simulink model "SpeedgoatCANOpen2Buses100us"  (R2018b)
settings: Solver=FixedStepDiscrete  StartTime=0.0  StopTime=inf  FixedStep=0.0001  RelTol=1e-3  EnableMultiTasking=on
libraries: slrtlib x6, speedgoatlib_IO691 x5, simulink x3, dspstat3 x2, cstblocks x1
(part 1 of 2)
settings Model: DataDictionary=Trike_dictionary.sldd  SimulationMode=external  Creator=Venqo  LastModifiedBy=Venqo
settings SolverCC: ConcurrentTasks=on  AutoInsertRateTranBlk=on
settings DataIOCC: SaveFormat=StructureWithTime
settings OptimizationCC: BlockReduction=off  OptimizeBlockIOStorage=off  BufferReuse=off  GlobalBufferReuse=off  ExpressionFolding=off  LocalBlockOutputs=off  RollThreshold=10  OptimizeDataStoreBuffers=off  BusAssignmentInplaceUpdate=off
settings DebuggingCC: ParameterOverflowMsg=none
settings HardwareCC: ProdBitPerPointer=32  ProdBitPerSizeT=32  ProdBitPerPtrDiffT=32  ProdLargestAtomicFloat=None  ProdWordSize=32  ProdLongLongMode=on  ProdHWDeviceType=Generic->32-bit x86 compatible
settings SFSimCC: SimAnalyzeCustomCode=on
settings SFSimCC: SimCustomHeaderCode=|
  | #include "CANOpenSlave.h"
  | #include "CANOpenSlaveAPT.h"
settings SFSimCC: SimCustomInitializer=|
  | CANOpenSlave_ResetCommunication();
  | CANOpenSlave_ResetCommunication_APT();
settings SFSimCC: SimUserSources=|
  | CANOpenSlave.c
  | CANOpenSlaveAPT.c
settings RTWCC: SystemTargetFile=slrt.tlc  TemplateMakefile=slrt_default_tmf  Description=Simulink Real-Time  CodeExecutionProfiling=on  RTWCompilerOptimization=on
settings RTWCC: CustomHeaderCode=|
  | #include "CANOpenSlave.h"
  | #include "CANOpenSlaveAPT.h"
settings RTWCC: CustomSource=|
  | CANOpenSlave.c
  | CANOpenSlaveAPT.c
settings RTWCC: CustomInitializer=|
  | CANOpenSlave_ResetCommunication();
  | CANOpenSlave_ResetCommunication_APT();
settings SimulinkRealTimeCC: InferredTypesCompatibility=on  SupportVariableSizeSignals=on  PreserveStateflowLocalDataDimensions=off  RL32LogTETModifier=off  RL32LogBufSizeModifier=140000  xPCConcurrentTasks=on

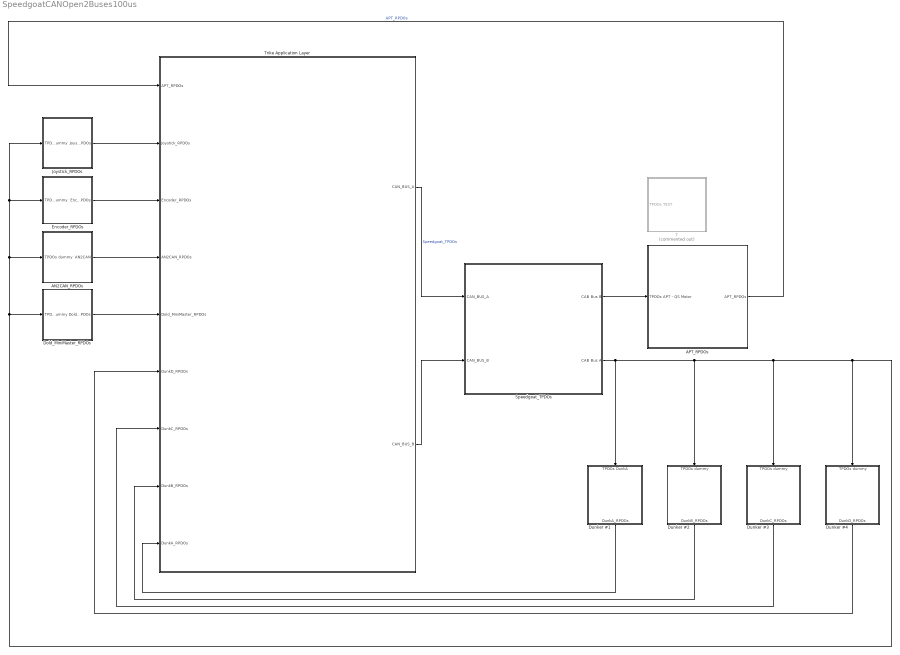
== system SpeedgoatCANOpen2Buses100us ==
  AN2CAN_RPDOs : Subsystem
      mask Display: image('Img\mcan_box_4xi.png');
  APT_RPDOs : Subsystem
      mask Display: image('Img\aptqsmotor.png');
  Dold_MiniMaster_RPDOs : Subsystem
      mask Display: image('C:\Users\Venqo\Desktop\SpeedGoat\Applications\Trike_git\Trike_SpeedGoat_algo\Img\dold - Copy.png');
  Dunker #1 : Subsystem
      mask Display: image('Img\dunk.png');
  Dunker #2 : Subsystem
      mask Display: image('Img\dunk.png');
  Dunker #3 : Subsystem
      mask Display: image('Img\dunk.png');
  Dunker #4 : Subsystem
      mask Display: image('Img\dunk.png');
  Encoder_RPDOs : Subsystem
      mask Display: image('Img\WDGA_Encoder.PNG');
  Joystick_RPDOs : Subsystem
      mask Display: image('Img\joystick.png');
  Speedgoat_TPDOs : Subsystem
      mask Display: image('Img\speedgoat.png');
  T : Subsystem  Commented=on
  Trike Application Layer : Subsystem
      mask Display: image('Img\trike.png');
  wires:
  Joystick_RPDOs/1(Joystick_RPDOs) -> Trike Application Layer/2(Joystick_RPDOs)
  Trike Application Layer/1(CAN_BUS_A) -> Speedgoat_TPDOs/1(CAN_BUS_A)  "Speedgoat_TPDOs"
  Dunker #1/1(DunkA_RPDOs) -> Trike Application Layer/9(DunkA_RPDOs)
  Encoder_RPDOs/1(Encoder_RPDOs) -> Trike Application Layer/3(Encoder_RPDOs)
  Dunker #2/1(DunkB_RPDOs) -> Trike Application Layer/8(DunkB_RPDOs)
  Dunker #3/1(DunkC_RPDOs) -> Trike Application Layer/7(DunkC_RPDOs)
  Dunker #4/1(DunkD_RPDOs) -> Trike Application Layer/6(DunkD_RPDOs)
  AN2CAN_RPDOs/1(AN2CAN) -> Trike Application Layer/4(AN2CAN_RPDOs)
  Speedgoat_TPDOs/1(CAB Bus B) -> APT_RPDOs/1("TPDOs APT - QS Motor ")
  APT_RPDOs/1(APT_RPDOs) -> Trike Application Layer/1(APT_RPDOs)  "APT_RPDOs"
  Trike Application Layer/2(CAN_BUS_B) -> Speedgoat_TPDOs/2(CAN_BUS_B)
  Dold_MiniMaster_RPDOs/1(Dold_RPDOs) -> Trike Application Layer/5(Dold_MiniMaster_RPDOs)
  Speedgoat_TPDOs/2("CAB Bus A ") -> Dold_MiniMaster_RPDOs/1(TPDOs dummy), Joystick_RPDOs/1(TPDOs dummy), Encoder_RPDOs/1(TPDOs dummy), AN2CAN_RPDOs/1(TPDOs dummy), Dunker #4/1(TPDOs dummy), Dunker #3/1(TPDOs dummy), Dunker #2/1(TPDOs dummy), Dunker #1/1(TPDOs DunkA)

== system SpeedgoatCANOpen2Buses100us/AN2CAN_RPDOs ==
  TPDOs dummy : Inport
  Bus Creator : BusCreator  Inputs=4  OutDataTypeStr=Bus: AN2CAN_conv
  "RPDOs from AN2CAN " : S-Function  InitFcn=try, set_param(gcb,'FunctionName','RPDOs_from_AN2CANConv'), end  FunctionName=RPDOs_from_AN2CANConv  SFunctionModules=RPDOs_from_AN2CANConv_wrapper  SFunctionDeploymentMode=off  EnableBusSupport=off  mask(S-Function Builder){}
      mask help: Simulink:masks:SFunctionBuilder_MD
      mask init:
      | val = [[.9  0.75 0.75 1 1 .9 .9 1]',[1 1 0.75 0.75 .9 .9 1 .9]'];try , sys = get_param(gcb,'SfunBuilderFcnName');if isempty(sys), sys = get_param(gcb,'FunctionName'); end,catch, sys = get_param(gcb,'FunctionName'); end
      settings: CopyFcn=set_param(gcbh,'LinkStatus','none')  PreSaveFcn=try, set_param(gcb,'FunctionName','RPDOs_from_AN2CANConv'), end  OpenFcn=sfunctionwizard(gcbh)
      mask Display: plot(val(:,1),val(:,2)),disp(sys), port_label('output',1,'Channel_AN1'), port_label('output',2,'Channel_AN2'), port_label('output',3,'Channel_AN3'), port_label('output',4,'Channel_AN4')
  AN2CAN : Outport  OutDataTypeStr=Bus: AN2CAN_conv
  wires:
  Bus Creator/1 -> AN2CAN/1
  "RPDOs from AN2CAN "/4 -> Bus Creator/4  "Channel_AN4"
  "RPDOs from AN2CAN "/3 -> Bus Creator/3  "Channel_AN3"
  "RPDOs from AN2CAN "/1 -> Bus Creator/1  "Channel_AN1"
  "RPDOs from AN2CAN "/2 -> Bus Creator/2  "Channel_AN2"

== system SpeedgoatCANOpen2Buses100us/APT_RPDOs ==
  "TPDOs APT - QS Motor " : Inport  OutDataTypeStr=Bus: Speedgoat_TPDOs
  Bus Creator : BusCreator  Inputs=8  OutDataTypeStr=Bus: APT_RPDOs
  Bus Selector : BusSelector  OutputSignals=APT_TPDO_ControlWord,APT_TPDO_PedalPosition,APT_TPDO_Heartbeat
  RPDOs from APT : S-Function  InitFcn=try, set_param(gcb,'FunctionName','RPDOs_from_APT'), end  FunctionName=RPDOs_from_APT  SFunctionModules=RPDOs_from_APT_wrapper  SFunctionDeploymentMode=off  EnableBusSupport=off  mask(S-Function Builder){}
      mask help: Simulink:masks:SFunctionBuilder_MD
      mask init: same as SpeedgoatCANOpen2Buses100us/AN2CAN_RPDOs/RPDOs from AN2CAN 
      settings: CopyFcn=set_param(gcbh,'LinkStatus','none')  PreSaveFcn=try, set_param(gcb,'FunctionName','RPDOs_from_APT'), end  OpenFcn=sfunctionwizard(gcbh)
      mask Display: plot(val(:,1),val(:,2)),disp(sys), port_label('output',1,'StatusWord'), port_label('output',2,'PhaseCurrent'), port_label('output',3,'Speed'), port_label('output',4,'BusVoltage'), port_label('output',5,'MotorTemp'), port_label('output',6,'APTTemp'), port_label('output',7,'ErrStatus'), port_label('output',8,'Direction')
  TPDOs from Speedgoat to APT : S-Function  InitFcn=try, set_param(gcb,'FunctionName','TPDOs_to_APT'), end  FunctionName=TPDOs_to_APT  SFunctionModules=TPDOs_to_APT_wrapper  SFunctionDeploymentMode=off  EnableBusSupport=off  mask(S-Function Builder){}
      mask help: Simulink:masks:SFunctionBuilder_MD
      mask init: same as SpeedgoatCANOpen2Buses100us/AN2CAN_RPDOs/RPDOs from AN2CAN 
      settings: CopyFcn=set_param(gcbh,'LinkStatus','none')  PreSaveFcn=try, set_param(gcb,'FunctionName','TPDOs_to_APT'), end  OpenFcn=sfunctionwizard(gcbh)
      mask Display: plot(val(:,1),val(:,2)),disp(sys), port_label('input',1,'APT_ControlWord'), port_label('input',2,'APT_PedalPosition'), port_label('input',3,'APT_HeartBeat')
  APT_RPDOs : Outport  OutDataTypeStr=Bus: APT_RPDOs
  wires:
  Bus Creator/1 -> APT_RPDOs/1
  RPDOs from APT/8 -> Bus Creator/8  "APT_Direction"
  RPDOs from APT/2 -> Bus Creator/2  "APT_PhaseCurrent"
  RPDOs from APT/6 -> Bus Creator/6  "APT_Temp"
  RPDOs from APT/3 -> Bus Creator/3  "APT_Speed"
  RPDOs from APT/1 -> Bus Creator/1  "APT_StatusWord"
  RPDOs from APT/5 -> Bus Creator/5  "APT_MotorTemp"
  RPDOs from APT/7 -> Bus Creator/7  "APT_ErrStatus"
  RPDOs from APT/4 -> Bus Creator/4  "APT_BusVoltage"
  "TPDOs APT - QS Motor "/1 -> Bus Selector/1
  Bus Selector/1 -> TPDOs from Speedgoat to APT/1  "<APT_TPDO_ControlWord>"
  Bus Selector/2 -> TPDOs from Speedgoat to APT/2  "<APT_TPDO_PedalPosition>"
  Bus Selector/3 -> TPDOs from Speedgoat to APT/3  "<APT_TPDO_Heartbeat>"

== system SpeedgoatCANOpen2Buses100us/Dold_MiniMaster_RPDOs ==
  TPDOs dummy : Inport
  Bus Creator : BusCreator  Inputs=1  OutDataTypeStr=Bus: Dold_RPDOs
  Constant : Constant  OutDataTypeStr=uint8
  Dold_RPDOs : Outport  OutDataTypeStr=Bus: Dold_RPDOs
  wires:
  Bus Creator/1 -> Dold_RPDOs/1
  Constant/1 -> Bus Creator/1  "Enable"

== system SpeedgoatCANOpen2Buses100us/Dunker #1 ==
  TPDOs DunkA : Inport  OutDataTypeStr=Bus: Speedgoat_TPDOs
  Bus Creator : BusCreator  Inputs=2  OutDataTypeStr=Bus: Dunk_RPDOs
  Bus Selector : BusSelector  OutputSignals=DunkA_TPDO_ClearError,DunkA_TPDO_DeviceMode,DunkA_TPDO_PowerEnable,DunkA_TPDO_BrakeCtrl,DunkA_TPDO_DesiredCurrent
  RPDOs from Dunker #1 : S-Function  InitFcn=try, set_param(gcb,'FunctionName','RPDOs_from_DunkA'), end  FunctionName=RPDOs_from_DunkA  SFunctionModules=RPDOs_from_DunkA_wrapper  SFunctionDeploymentMode=off  EnableBusSupport=off  mask(S-Function Builder){}
      mask help: Simulink:masks:SFunctionBuilder_MD
      mask init: same as SpeedgoatCANOpen2Buses100us/AN2CAN_RPDOs/RPDOs from AN2CAN 
      settings: CopyFcn=set_param(gcbh,'LinkStatus','none')  PreSaveFcn=try, set_param(gcb,'FunctionName','RPDOs_from_DunkA'), end  OpenFcn=sfunctionwizard(gcbh)
      mask Display: plot(val(:,1),val(:,2)),disp(sys), port_label('output',1,'ActualCurrent'), port_label('output',2,'ActualVelocity')
  TPDOs from Speedgoat to Dunker #1 : S-Function  InitFcn=try, set_param(gcb,'FunctionName','TPDOs_to_DunkA'), end  FunctionName=TPDOs_to_DunkA  SFunctionModules=TPDOs_to_DunkA_wrapper  SFunctionDeploymentMode=off  EnableBusSupport=off  mask(S-Function Builder){}
      mask help: Simulink:masks:SFunctionBuilder_MD
      mask init: same as SpeedgoatCANOpen2Buses100us/AN2CAN_RPDOs/RPDOs from AN2CAN 
      settings: CopyFcn=set_param(gcbh,'LinkStatus','none')  PreSaveFcn=try, set_param(gcb,'FunctionName','TPDOs_to_DunkA'), end  OpenFcn=sfunctionwizard(gcbh)
      mask Display: plot(val(:,1),val(:,2)),disp(sys), port_label('input',1,'ClearError'), port_label('input',2,'DeviceMode'), port_label('input',3,'PowerEnable'), port_label('input',4,'BrakeCtrl'), port_label('input',5,'DesiredCurrent')
  DunkA_RPDOs : Outport  OutDataTypeStr=Bus: Dunk_RPDOs
  wires:
  Bus Creator/1 -> DunkA_RPDOs/1
  RPDOs from Dunker #1/1 -> Bus Creator/1  "DunkA_ActualCurrent"
  RPDOs from Dunker #1/2 -> Bus Creator/2  "DunkA_ActualVelocity"
  Bus Selector/5 -> TPDOs from Speedgoat to Dunker #1/5  "<DunkA_TPDO_DesiredCurrent>"
  Bus Selector/1 -> TPDOs from Speedgoat to Dunker #1/1  "<DunkA_TPDO_ClearError>"
  Bus Selector/3 -> TPDOs from Speedgoat to Dunker #1/3  "<DunkA_TPDO_PowerEnable>"
  Bus Selector/4 -> TPDOs from Speedgoat to Dunker #1/4  "<DunkA_TPDO_BrakeCtrl>"
  Bus Selector/2 -> TPDOs from Speedgoat to Dunker #1/2  "<DunkA_TPDO_DeviceMode>"
  TPDOs DunkA/1 -> Bus Selector/1

== system SpeedgoatCANOpen2Buses100us/Dunker #2 ==
  TPDOs dummy : Inport  OutDataTypeStr=Bus: Speedgoat_TPDOs
  Bus Creator : BusCreator  Inputs=2  OutDataTypeStr=Bus: Dunk_RPDOs
  Bus Selector : BusSelector  OutputSignals=DunkB_TPDO_ClearError,DunkB_TPDO_DeviceMode,DunkB_TPDO_PowerEnable,DunkB_TPDO_BrakeCtrl,DunkB_TPDO_DesiredCurrent
  RPDOs from Dunker #1 : S-Function  InitFcn=try, set_param(gcb,'FunctionName','RPDOs_from_DunkB'), end  FunctionName=RPDOs_from_DunkB  SFunctionModules=RPDOs_from_DunkB_wrapper  SFunctionDeploymentMode=off  EnableBusSupport=off  mask(S-Function Builder){}
      mask help: Simulink:masks:SFunctionBuilder_MD
      mask init: same as SpeedgoatCANOpen2Buses100us/AN2CAN_RPDOs/RPDOs from AN2CAN 
      settings: CopyFcn=set_param(gcbh,'LinkStatus','none')  PreSaveFcn=try, set_param(gcb,'FunctionName','RPDOs_from_DunkB'), end  OpenFcn=sfunctionwizard(gcbh)
      mask Display: plot(val(:,1),val(:,2)),disp(sys), port_label('output',1,'ActualCurrent'), port_label('output',2,'ActualVelocity')
  TPDOs from Speedgoat to Dunker #1 : S-Function  InitFcn=try, set_param(gcb,'FunctionName','TPDOs_to_DunkB'), end  FunctionName=TPDOs_to_DunkB  SFunctionModules=TPDOs_to_DunkB_wrapper  SFunctionDeploymentMode=off  EnableBusSupport=off  mask(S-Function Builder){}
      mask help: Simulink:masks:SFunctionBuilder_MD
      mask init: same as SpeedgoatCANOpen2Buses100us/AN2CAN_RPDOs/RPDOs from AN2CAN 
      settings: CopyFcn=set_param(gcbh,'LinkStatus','none')  PreSaveFcn=try, set_param(gcb,'FunctionName','TPDOs_to_DunkB'), end  OpenFcn=sfunctionwizard(gcbh)
      mask Display: plot(val(:,1),val(:,2)),disp(sys), port_label('input',1,'ClearError'), port_label('input',2,'DeviceMode'), port_label('input',3,'PowerEnable'), port_label('input',4,'BrakeCtrl'), port_label('input',5,'DesiredCurrent')
  DunkB_RPDOs : Outport  OutDataTypeStr=Bus: Dunk_RPDOs
  wires:
  TPDOs dummy/1 -> Bus Selector/1
  Bus Selector/2 -> TPDOs from Speedgoat to Dunker #1/2  "<DunkB_TPDO_DeviceMode>"
  Bus Selector/4 -> TPDOs from Speedgoat to Dunker #1/4  "<DunkB_TPDO_BrakeCtrl>"
  Bus Selector/3 -> TPDOs from Speedgoat to Dunker #1/3  "<DunkB_TPDO_PowerEnable>"
  Bus Selector/1 -> TPDOs from Speedgoat to Dunker #1/1  "<DunkB_TPDO_ClearError>"
  Bus Selector/5 -> TPDOs from Speedgoat to Dunker #1/5  "<DunkB_TPDO_DesiredCurrent>"
  RPDOs from Dunker #1/2 -> Bus Creator/2  "DunkB_ActualVelocity"
  RPDOs from Dunker #1/1 -> Bus Creator/1  "DunkB_ActualCurrent"
  Bus Creator/1 -> DunkB_RPDOs/1

== system SpeedgoatCANOpen2Buses100us/Dunker #3 ==
  TPDOs dummy : Inport  OutDataTypeStr=Bus: Speedgoat_TPDOs
  Bus Creator : BusCreator  Inputs=2  OutDataTypeStr=Bus: Dunk_RPDOs
  Bus Selector : BusSelector  OutputSignals=DunkC_TPDO_ClearError,DunkC_TPDO_DeviceMode,DunkC_TPDO_PowerEnable,DunkC_TPDO_BrakeCtrl,DunkC_TPDO_DesiredCurrent
  Gain : Gain  Gain=-1
  RPDOs from Dunker #1 : S-Function  InitFcn=try, set_param(gcb,'FunctionName','RPDOs_from_DunkC'), end  FunctionName=RPDOs_from_DunkC  SFunctionModules=RPDOs_from_DunkC_wrapper  SFunctionDeploymentMode=off  EnableBusSupport=off  mask(S-Function Builder){}
      mask help: Simulink:masks:SFunctionBuilder_MD
      mask init: same as SpeedgoatCANOpen2Buses100us/AN2CAN_RPDOs/RPDOs from AN2CAN 
      settings: CopyFcn=set_param(gcbh,'LinkStatus','none')  PreSaveFcn=try, set_param(gcb,'FunctionName','RPDOs_from_DunkC'), end  OpenFcn=sfunctionwizard(gcbh)
      mask Display: plot(val(:,1),val(:,2)),disp(sys), port_label('output',1,'ActualCurrent'), port_label('output',2,'ActualVelocity')
  TPDOs from Speedgoat to Dunker #1 : S-Function  InitFcn=try, set_param(gcb,'FunctionName','TPDOs_to_DunkC'), end  FunctionName=TPDOs_to_DunkC  SFunctionModules=TPDOs_to_DunkC_wrapper  SFunctionDeploymentMode=off  EnableBusSupport=off  mask(S-Function Builder){}
      mask help: Simulink:masks:SFunctionBuilder_MD
      mask init: same as SpeedgoatCANOpen2Buses100us/AN2CAN_RPDOs/RPDOs from AN2CAN 
      settings: CopyFcn=set_param(gcbh,'LinkStatus','none')  PreSaveFcn=try, set_param(gcb,'FunctionName','TPDOs_to_DunkC'), end  OpenFcn=sfunctionwizard(gcbh)
      mask Display: plot(val(:,1),val(:,2)),disp(sys), port_label('input',1,'ClearError'), port_label('input',2,'DeviceMode'), port_label('input',3,'PowerEnable'), port_label('input',4,'BrakeCtrl'), port_label('input',5,'DesiredCurrent')
  Terminator : Terminator
  DunkC_RPDOs : Outport  OutDataTypeStr=Bus: Dunk_RPDOs
  wires:
  Bus Creator/1 -> DunkC_RPDOs/1
  RPDOs from Dunker #1/1 -> Gain/1, Bus Creator/1  "DunkC_ActualCurrent"
  RPDOs from Dunker #1/2 -> Bus Creator/2  "DunkC_ActualVelocity"
  Bus Selector/5 -> TPDOs from Speedgoat to Dunker #1/5  "<DunkC_TPDO_DesiredCurrent>"
  Bus Selector/1 -> TPDOs from Speedgoat to Dunker #1/1  "<DunkC_TPDO_ClearError>"
  Bus Selector/2 -> TPDOs from Speedgoat to Dunker #1/2  "<DunkC_TPDO_DeviceMode>"
  Bus Selector/4 -> TPDOs from Speedgoat to Dunker #1/4  "<DunkC_TPDO_BrakeCtrl>"
  Bus Selector/3 -> TPDOs from Speedgoat to Dunker #1/3  "<DunkC_TPDO_PowerEnable>"
  TPDOs dummy/1 -> Bus Selector/1
  Gain/1 -> Terminator/1  "DunkC_ActualCurrent_Inv"

== system SpeedgoatCANOpen2Buses100us/Dunker #4 ==
  TPDOs dummy : Inport  OutDataTypeStr=Bus: Speedgoat_TPDOs
  Bus Creator : BusCreator  Inputs=2  OutDataTypeStr=Bus: Dunk_RPDOs
  Bus Selector : BusSelector  OutputSignals=DunkD_TPDO_ClearError,DunkD_TPDO_DeviceMode,DunkD_TPDO_PowerEnable,DunkD_TPDO_BrakeCtrl,DunkD_TPDO_DesiredCurrent
  RPDOs from Dunker #1 : S-Function  InitFcn=try, set_param(gcb,'FunctionName','RPDOs_from_DunkD'), end  FunctionName=RPDOs_from_DunkD  SFunctionModules=RPDOs_from_DunkD_wrapper  SFunctionDeploymentMode=off  EnableBusSupport=off  mask(S-Function Builder){}
      mask help: Simulink:masks:SFunctionBuilder_MD
      mask init: same as SpeedgoatCANOpen2Buses100us/AN2CAN_RPDOs/RPDOs from AN2CAN 
      settings: CopyFcn=set_param(gcbh,'LinkStatus','none')  PreSaveFcn=try, set_param(gcb,'FunctionName','RPDOs_from_DunkD'), end  OpenFcn=sfunctionwizard(gcbh)
      mask Display: plot(val(:,1),val(:,2)),disp(sys), port_label('output',1,'ActualCurrent'), port_label('output',2,'ActualVelocity')
  TPDOs from Speedgoat to Dunker #1 : S-Function  InitFcn=try, set_param(gcb,'FunctionName','TPDOs_to_DunkD'), end  FunctionName=TPDOs_to_DunkD  SFunctionModules=TPDOs_to_DunkD_wrapper  SFunctionDeploymentMode=off  EnableBusSupport=off  mask(S-Function Builder){}
      mask help: Simulink:masks:SFunctionBuilder_MD
      mask init: same as SpeedgoatCANOpen2Buses100us/AN2CAN_RPDOs/RPDOs from AN2CAN 
      settings: CopyFcn=set_param(gcbh,'LinkStatus','none')  PreSaveFcn=try, set_param(gcb,'FunctionName','TPDOs_to_DunkD'), end  OpenFcn=sfunctionwizard(gcbh)
      mask Display: plot(val(:,1),val(:,2)),disp(sys), port_label('input',1,'ClearError'), port_label('input',2,'DeviceMode'), port_label('input',3,'PowerEnable'), port_label('input',4,'BrakeCtrl'), port_label('input',5,'DesiredCurrent')
  DunkD_RPDOs : Outport  OutDataTypeStr=Bus: Dunk_RPDOs
  wires:
  TPDOs dummy/1 -> Bus Selector/1
  Bus Selector/2 -> TPDOs from Speedgoat to Dunker #1/2  "<DunkD_TPDO_DeviceMode>"
  Bus Selector/4 -> TPDOs from Speedgoat to Dunker #1/4  "<DunkD_TPDO_BrakeCtrl>"
  Bus Selector/3 -> TPDOs from Speedgoat to Dunker #1/3  "<DunkD_TPDO_PowerEnable>"
  Bus Selector/1 -> TPDOs from Speedgoat to Dunker #1/1  "<DunkD_TPDO_ClearError>"
  Bus Selector/5 -> TPDOs from Speedgoat to Dunker #1/5  "<DunkD_TPDO_DesiredCurrent>"
  RPDOs from Dunker #1/2 -> Bus Creator/2  "DunkD_ActualVelocity"
  RPDOs from Dunker #1/1 -> Bus Creator/1  "DunkD_ActualCurrent"
  Bus Creator/1 -> DunkD_RPDOs/1

== system SpeedgoatCANOpen2Buses100us/Encoder_RPDOs ==
  TPDOs dummy : Inport
  Bus Creator : BusCreator  Inputs=2  OutDataTypeStr=Bus: Encoder_RPDOs
  RPDOs from Encoder : S-Function  InitFcn=try, set_param(gcb,'FunctionName','RPDOs_from_Encoder'), end  FunctionName=RPDOs_from_Encoder  SFunctionModules=RPDOs_from_Encoder_wrapper  SFunctionDeploymentMode=off  EnableBusSupport=off  mask(S-Function Builder){}
      mask help: Simulink:masks:SFunctionBuilder_MD
      mask init: same as SpeedgoatCANOpen2Buses100us/AN2CAN_RPDOs/RPDOs from AN2CAN 
      settings: CopyFcn=set_param(gcbh,'LinkStatus','none')  PreSaveFcn=try, set_param(gcb,'FunctionName','RPDOs_from_Encoder'), end  OpenFcn=sfunctionwizard(gcbh)
      mask Display: plot(val(:,1),val(:,2)),disp(sys), port_label('output',1,'Encoder_Actual_Position'), port_label('output',2,'Encoder_Stored_Position')
  Encoder_RPDOs : Outport  OutDataTypeStr=Bus: Encoder_RPDOs
  wires:
  RPDOs from Encoder/1 -> Bus Creator/1  "Encoder_Actual_Position"
  RPDOs from Encoder/2 -> Bus Creator/2  "Encoder_Stored_Position"
  Bus Creator/1 -> Encoder_RPDOs/1

== system SpeedgoatCANOpen2Buses100us/Joystick_RPDOs ==
  TPDOs dummy : Inport
  Bus Creator : BusCreator  Inputs=3  OutDataTypeStr=Bus: Joystick_RPDOs
  RPDOs from Joystick : S-Function  InitFcn=try, set_param(gcb,'FunctionName','RPDOs_from_Joystick'), end  FunctionName=RPDOs_from_Joystick  SFunctionModules=RPDOs_from_Joystick_wrapper  SFunctionDeploymentMode=off  EnableBusSupport=off  mask(S-Function Builder){}
      mask help: Simulink:masks:SFunctionBuilder_MD
      mask init: same as SpeedgoatCANOpen2Buses100us/AN2CAN_RPDOs/RPDOs from AN2CAN 
      settings: CopyFcn=set_param(gcbh,'LinkStatus','none')  PreSaveFcn=try, set_param(gcb,'FunctionName','RPDOs_from_Joystick'), end  OpenFcn=sfunctionwizard(gcbh)
      mask Display: plot(val(:,1),val(:,2)),disp(sys), port_label('output',1,'ButtonsStatus'), port_label('output',2,'LongCmd'), port_label('output',3,'LatCmd')
  Joystick_RPDOs : Outport  OutDataTypeStr=Bus: Joystick_RPDOs
  wires:
  RPDOs from Joystick/3 -> Bus Creator/3  "Joystick_LatCmd"
  RPDOs from Joystick/2 -> Bus Creator/2  "Joystick_LongCmd"
  RPDOs from Joystick/1 -> Bus Creator/1  "Joystick_ButtonsStatus"
  Bus Creator/1 -> Joystick_RPDOs/1

== system SpeedgoatCANOpen2Buses100us/Speedgoat_TPDOs ==
  CAN_BUS_A : Inport  OutDataTypeStr=Bus: CAN_BUS_A
  CAN_BUS_B : Inport  Port=2  OutDataTypeStr=Bus: CAN_BUS_B
  CAN Bus Communication : Subsystem
  Subsystem : Subsystem
  CAB Bus B : Outport  OutDataTypeStr=Bus: Speedgoat_TPDOs
  "CAB Bus A " : Outport  Port=2  OutDataTypeStr=Bus: Speedgoat_TPDOs
  wires:
  Subsystem/1(SpeedGoat) -> "CAB Bus A "/1, CAB Bus B/1
  CAN_BUS_B/1 -> Subsystem/2(CAN_BUS_B)
  CAN_BUS_A/1 -> Subsystem/1(CAN_BUS_A)

== system SpeedgoatCANOpen2Buses100us/T ==
  TPDOs TEST : Inport  OutDataTypeStr=Bus: Speedgoat_TPDOs
  Bus Selector : BusSelector  OutputSignals=AN_01,AN_02,AN_03,AN_04
  TPDOs from Speedgoat to Dunker #1 : S-Function  InitFcn=try, set_param(gcb,'FunctionName','TPDOs_TEST'), end  FunctionName=TPDOs_TEST  SFunctionModules=TPDOs_TEST_wrapper  SFunctionDeploymentMode=off  EnableBusSupport=off  mask(S-Function Builder){}
      mask help: Simulink:masks:SFunctionBuilder_MD
      mask init: same as SpeedgoatCANOpen2Buses100us/AN2CAN_RPDOs/RPDOs from AN2CAN 
      settings: CopyFcn=set_param(gcbh,'LinkStatus','none')  PreSaveFcn=try, set_param(gcb,'FunctionName','TPDOs_TEST'), end  OpenFcn=sfunctionwizard(gcbh)
      mask Display: plot(val(:,1),val(:,2)),disp(sys), port_label('input',1,'AN1'), port_label('input',2,'AN2'), port_label('input',3,'AN3'), port_label('input',4,'AN4')
  wires:
  Bus Selector/1 -> TPDOs from Speedgoat to Dunker #1/1  "<AN_01>"
  Bus Selector/3 -> TPDOs from Speedgoat to Dunker #1/3  "<AN_03>"
  Bus Selector/4 -> TPDOs from Speedgoat to Dunker #1/4  "<AN_04>"
  Bus Selector/2 -> TPDOs from Speedgoat to Dunker #1/2  "<AN_02>"
  TPDOs TEST/1 -> Bus Selector/1

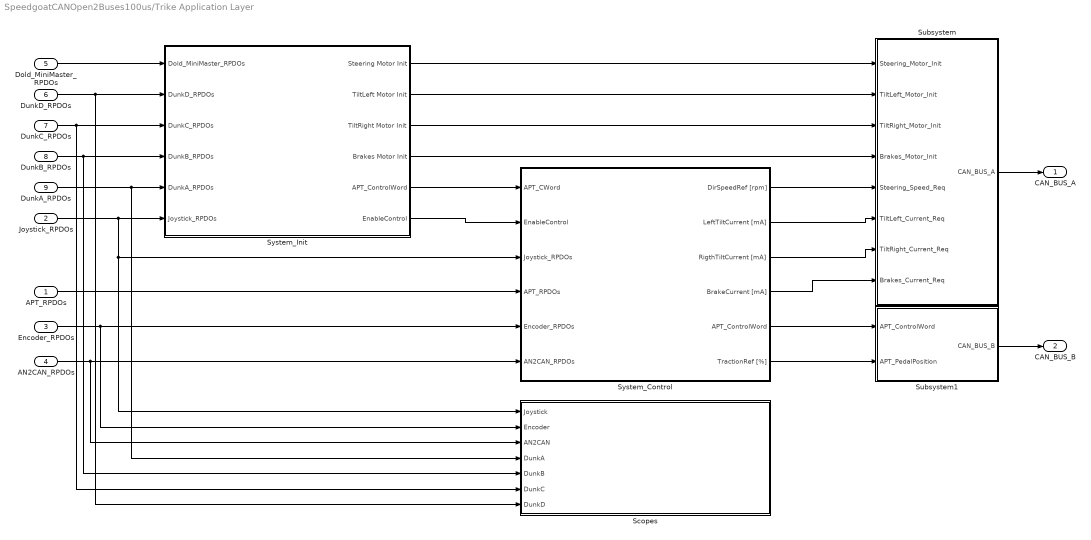
== system SpeedgoatCANOpen2Buses100us/Trike Application Layer ==
  APT_RPDOs : Inport  OutDataTypeStr=Bus: APT_RPDOs
  Joystick_RPDOs : Inport  Port=2  OutDataTypeStr=Bus: Joystick_RPDOs
  Encoder_RPDOs : Inport  Port=3  OutDataTypeStr=Bus: Encoder_RPDOs
  AN2CAN_RPDOs : Inport  Port=4  OutDataTypeStr=Bus: AN2CAN_conv
  Dold_MiniMaster_RPDOs : Inport  Port=5  OutDataTypeStr=Bus: Dold_RPDOs
  DunkD_RPDOs : Inport  Port=6  OutDataTypeStr=Bus: Dunk_RPDOs
  DunkC_RPDOs : Inport  Port=7  OutDataTypeStr=Bus: Dunk_RPDOs
  DunkB_RPDOs : Inport  Port=8  OutDataTypeStr=Bus: Dunk_RPDOs
  DunkA_RPDOs : Inport  Port=9  OutDataTypeStr=Bus: Dunk_RPDOs
  Scopes : Subsystem
  Subsystem : Subsystem
  Subsystem1 : Subsystem
  System_Control : Subsystem
  System_Init : Subsystem
  CAN_BUS_A : Outport  OutDataTypeStr=Bus: CAN_BUS_A
  CAN_BUS_B : Outport  Port=2  OutDataTypeStr=Bus: CAN_BUS_B
  wires:
  Subsystem/1(CAN_BUS_A) -> CAN_BUS_A/1
  System_Control/1(DirSpeedRef [rpm]) -> Subsystem/5(Steering_Speed_Req)
  System_Control/2(LeftTiltCurrent [mA]) -> Subsystem/6(TiltLeft_Current_Req)
  System_Control/3(RigthTiltCurrent [mA]) -> Subsystem/7(TiltRight_Current_Req)
  System_Control/4(BrakeCurrent [mA]) -> Subsystem/8(Brakes_Current_Req)
  Subsystem1/1(CAN_BUS_B) -> CAN_BUS_B/1
  System_Control/6(TractionRef [%]) -> Subsystem1/2(APT_PedalPosition)
  DunkA_RPDOs/1 -> System_Init/5(DunkA_RPDOs), Scopes/4(DunkA)
  DunkB_RPDOs/1 -> System_Init/4(DunkB_RPDOs), Scopes/5(DunkB)
  DunkC_RPDOs/1 -> System_Init/3(DunkC_RPDOs), Scopes/6(DunkC)
  DunkD_RPDOs/1 -> Scopes/7(DunkD), System_Init/2(DunkD_RPDOs)
  System_Init/1(Steering Motor Init) -> Subsystem/1(Steering_Motor_Init)
  System_Init/2(TiltLeft Motor Init) -> Subsystem/2(TiltLeft_Motor_Init)
  System_Init/3(TiltRight Motor Init) -> Subsystem/3(TiltRight_Motor_Init)
  System_Init/4(Brakes Motor Init) -> Subsystem/4(Brakes_Motor_Init)
  System_Control/5(APT_ControlWord) -> Subsystem1/1(APT_ControlWord)
  AN2CAN_RPDOs/1 -> Scopes/3(AN2CAN), System_Control/6(AN2CAN_RPDOs)
  Encoder_RPDOs/1 -> Scopes/2(Encoder), System_Control/5(Encoder_RPDOs)
  APT_RPDOs/1 -> System_Control/4(APT_RPDOs)
  System_Init/6(EnableControl) -> System_Control/2(EnableControl)
  Joystick_RPDOs/1 -> System_Init/6(Joystick_RPDOs), Scopes/1(Joystick), System_Control/3(Joystick_RPDOs)
  System_Init/5(APT_ControlWord) -> System_Control/1(APT_CWord)
  Dold_MiniMaster_RPDOs/1 -> System_Init/1(Dold_MiniMaster_RPDOs)

== system SpeedgoatCANOpen2Buses100us/Speedgoat_TPDOs/CAN Bus Communication ==
  "CAN Setup " : speedgoatlib_IO691/CAN Setup   moduletype=IO691  id=1  pciSlot=-1  chn1=CAN (HS)  chn2=CAN (HS)  chn3=Disabled  chn4=Disabled  initStruct=[]  termStruct=[]  ArbitrationbdrChn1=500 kBaud  ArbitrationManbdrChn1=[2,16,63,16]  FdbdrChn1=5.0 MBaud  FdManbdrChn1=[2,2,5,2]  ArbitrationbdrChn2=500 kBaud  ArbitrationManbdrChn2=[2,16,63,16]  FdbdrChn2=5.0 MBaud  FdManbdrChn2=[2,2,5,2]  ArbitrationbdrChn3=1.0 MBaud  ArbitrationManbdrChn3=[2,8,31,8]  FdbdrChn3=5.0 MBaud  FdManbdrChn3=[2,2,5,2]  ArbitrationbdrChn4=1.0 MBaud  ArbitrationManbdrChn4=[2,8,31,8]  FdbdrChn4=5.0 MBaud  FdManbdrChn4=[2,2,5,2]  moduleInitValues=[691 1 -1 -1]
      settings: SourceProductName=Simulink Real-Time: Speedgoat Library
  CANOpen Slave Protocol Stack - CAN Bus #1 (A) : Subsystem  mask{Ts=0.0001}
      mask prompts: Ts "Sample Time (s)"
      mask Display: disp('CANOpen Slave Stack')
  CANOpen Slave Protocol Stack - CAN Bus #2 (B) : Subsystem  mask{Ts=0.0001}
      mask prompts: Ts "Sample Time (s)"
      mask Display: disp('CANOpen Slave Stack')

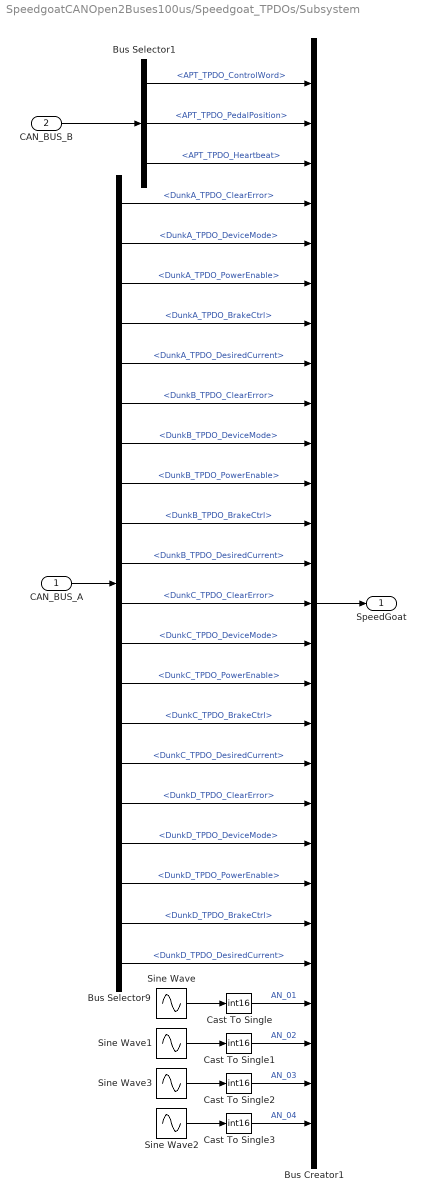
== system SpeedgoatCANOpen2Buses100us/Speedgoat_TPDOs/Subsystem ==
  CAN_BUS_A : Inport  OutDataTypeStr=Bus: CAN_BUS_A
  CAN_BUS_B : Inport  Port=2  OutDataTypeStr=Bus: CAN_BUS_B
  Bus Creator1 : BusCreator  Inputs=27  OutDataTypeStr=Bus: Speedgoat_TPDOs
  Bus Selector1 : BusSelector  OutputSignals=APT_TPDO_ControlWord,APT_TPDO_PedalPosition,APT_TPDO_Heartbeat
  Bus Selector9 : BusSelector  OutputSignals=DunkA_TPDO_ClearError,DunkA_TPDO_DeviceMode,DunkA_TPDO_PowerEnable,DunkA_TPDO_BrakeCtrl,DunkA_TPDO_DesiredCurrent,DunkB_TPDO_ClearError,DunkB_TPDO_DeviceMode,DunkB_TPDO_PowerEnable,DunkB_TPDO_BrakeCtrl,DunkB_TPDO_DesiredCurrent,DunkC_TPDO_ClearError,DunkC_TPDO_DeviceMode,DunkC_TPDO_PowerEnable,DunkC_TPDO_BrakeCtrl,DunkC_TPDO_DesiredCurrent,DunkD_TPDO_ClearError,DunkD_TPDO_DeviceMode,DunkD_TPDO_PowerEnable,DunkD_TPDO_BrakeCtrl,DunkD_TPDO_DesiredCurrent
  Cast To Single{,1..3} (4 alike) : DataTypeConversion  OutDataTypeStr=int16
  Sine Wave{,1..3} (4 alike) : Sin  Amplitude=5000  Bias=2500  Frequency=4  SampleTime=0
  SpeedGoat : Outport  OutDataTypeStr=Bus: Speedgoat_TPDOs
  wires:
  Bus Creator1/1 -> SpeedGoat/1
  CAN_BUS_A/1 -> Bus Selector9/1
  CAN_BUS_B/1 -> Bus Selector1/1
  Bus Selector1/1 -> Bus Creator1/1  "<APT_TPDO_ControlWord>"
  Bus Selector1/2 -> Bus Creator1/2  "<APT_TPDO_PedalPosition>"
  Bus Selector1/3 -> Bus Creator1/3  "<APT_TPDO_Heartbeat>"
  Bus Selector9/1 -> Bus Creator1/4  "<DunkA_TPDO_ClearError>"
  Bus Selector9/2 -> Bus Creator1/5  "<DunkA_TPDO_DeviceMode>"
  Bus Selector9/3 -> Bus Creator1/6  "<DunkA_TPDO_PowerEnable>"
  Bus Selector9/4 -> Bus Creator1/7  "<DunkA_TPDO_BrakeCtrl>"
  Bus Selector9/5 -> Bus Creator1/8  "<DunkA_TPDO_DesiredCurrent>"
  Bus Selector9/6 -> Bus Creator1/9  "<DunkB_TPDO_ClearError>"
  Bus Selector9/7 -> Bus Creator1/10  "<DunkB_TPDO_DeviceMode>"
  Bus Selector9/8 -> Bus Creator1/11  "<DunkB_TPDO_PowerEnable>"
  Bus Selector9/9 -> Bus Creator1/12  "<DunkB_TPDO_BrakeCtrl>"
  Bus Selector9/10 -> Bus Creator1/13  "<DunkB_TPDO_DesiredCurrent>"
  Bus Selector9/11 -> Bus Creator1/14  "<DunkC_TPDO_ClearError>"
  Bus Selector9/12 -> Bus Creator1/15  "<DunkC_TPDO_DeviceMode>"
  Bus Selector9/13 -> Bus Creator1/16  "<DunkC_TPDO_PowerEnable>"
  Bus Selector9/14 -> Bus Creator1/17  "<DunkC_TPDO_BrakeCtrl>"
  Bus Selector9/15 -> Bus Creator1/18  "<DunkC_TPDO_DesiredCurrent>"
  Bus Selector9/16 -> Bus Creator1/19  "<DunkD_TPDO_ClearError>"
  Bus Selector9/17 -> Bus Creator1/20  "<DunkD_TPDO_DeviceMode>"
  Bus Selector9/18 -> Bus Creator1/21  "<DunkD_TPDO_PowerEnable>"
  Bus Selector9/19 -> Bus Creator1/22  "<DunkD_TPDO_BrakeCtrl>"
  Bus Selector9/20 -> Bus Creator1/23  "<DunkD_TPDO_DesiredCurrent>"
  Sine Wave/1 -> Cast To Single/1
  Sine Wave1/1 -> Cast To Single1/1
  Sine Wave2/1 -> Cast To Single3/1
  Sine Wave3/1 -> Cast To Single2/1
  Cast To Single/1 -> Bus Creator1/24  "AN_01"
  Cast To Single1/1 -> Bus Creator1/25  "AN_02"
  Cast To Single2/1 -> Bus Creator1/26  "AN_03"
  Cast To Single3/1 -> Bus Creator1/27  "AN_04"

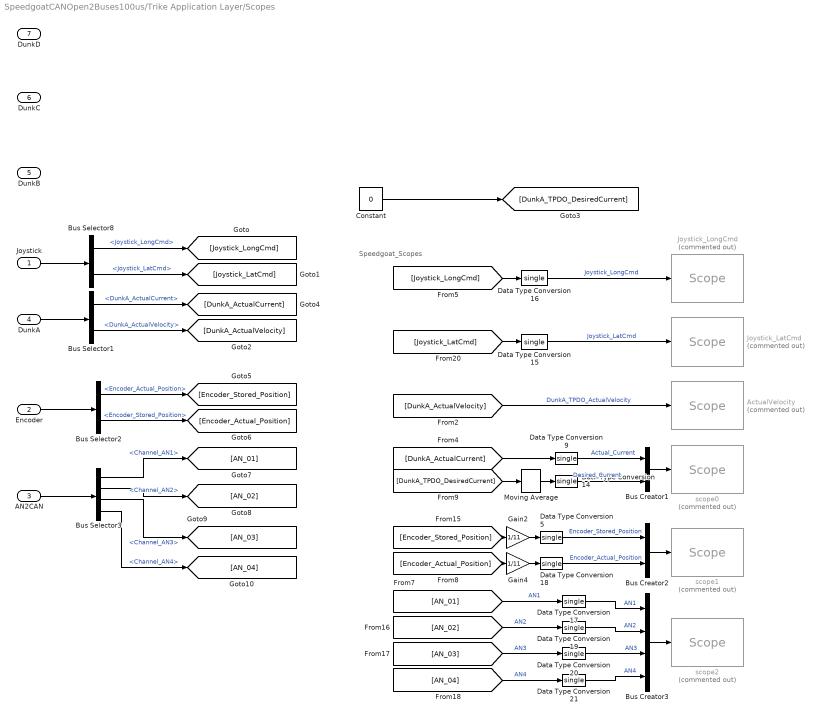
== system SpeedgoatCANOpen2Buses100us/Trike Application Layer/Scopes ==
  note: Speedgoat_Scopes
  Joystick : Inport
  Encoder : Inport  Port=2
  AN2CAN : Inport  Port=3
  DunkA : Inport  Port=4
  DunkB : Inport  Port=5
  DunkC : Inport  Port=6
  DunkD : Inport  Port=7
  ActualVelocity : slrtlib/Displays and Logging/Scope   Commented=on  scopeno=3  scopetype=Target  autostart=on  viewmode=Graphical sliding  formatstr='%15.6f'  grid=on  ylimits=[-3000,3000]  nosamples=30000  noprepostsamples=0  interleave=1  triggermode=FreeRun  triggersignal=1  trigsignalfromport=off  triggerlevel=0.0  triggerslope=Rising  triggerscope=1  triggersample=0  filename=data.dat  mode=Lazy  writesize=512  autorestart=off  dynamicfilemode=off  maxwritefilesize=512*1024^2
  Bus Creator1 : BusCreator  Inputs=2
  Bus Creator2 : BusCreator  Inputs=2
  Bus Creator3 : BusCreator  Inputs=4
  Bus Selector1 : BusSelector  OutputSignals=DunkA_ActualCurrent,DunkA_ActualVelocity
  Bus Selector2 : BusSelector  OutputSignals=Encoder_Actual_Position,Encoder_Stored_Position
  Bus Selector3 : BusSelector  OutputSignals=Channel_AN1,Channel_AN2,Channel_AN3,Channel_AN4
  Bus Selector8 : BusSelector  OutputSignals=Joystick_LongCmd,Joystick_LatCmd
  Constant : Constant  Value=0
  Data Type Conversion{5,9,14..21} (10 alike) : DataTypeConversion  OutDataTypeStr=single
  Gain2 : Gain  Gain=1/11
  Gain4 : Gain  Gain=1/11
  Joystick_LatCmd : slrtlib/Displays and Logging/Scope   Commented=on  scopeno=2  scopetype=Target  autostart=on  viewmode=Graphical sliding  formatstr='%15.6f'  grid=on  ylimits=[-300,300]  nosamples=30000  noprepostsamples=0  interleave=1  triggermode=FreeRun  triggersignal=1  trigsignalfromport=off  triggerlevel=0.0  triggerslope=Rising  triggerscope=1  triggersample=0  filename=data.dat  mode=Lazy  writesize=512  autorestart=off  dynamicfilemode=off  maxwritefilesize=512*1024^2
  Joystick_LongCmd : slrtlib/Displays and Logging/Scope   Commented=on  scopeno=1  scopetype=Target  autostart=on  viewmode=Graphical sliding  formatstr='%15.6f'  grid=on  ylimits=[-300,300]  nosamples=30000  noprepostsamples=0  interleave=1  triggermode=FreeRun  triggersignal=1  trigsignalfromport=off  triggerlevel=0.0  triggerslope=Rising  triggerscope=1  triggersample=0  filename=data.dat  mode=Lazy  writesize=512  autorestart=off  dynamicfilemode=off  maxwritefilesize=512*1024^2
  Moving Average : dspstat3/Moving Average  Method=Sliding window  ForgettingFactorPort=off  SpecifyWindowLength=on  WindowLength=50  ForgettingFactor=0.9  SimulateUsing=Code generation
  scope0 : slrtlib/Displays and Logging/Scope   Commented=on  scopeno=4  scopetype=Target  autostart=on  viewmode=Graphical sliding  formatstr='%15.6f'  grid=on  ylimits=[-10000,10000]  nosamples=30000  noprepostsamples=0  interleave=1  triggermode=FreeRun  triggersignal=1  trigsignalfromport=off  triggerlevel=0.0  triggerslope=Rising  triggerscope=1  triggersample=0  filename=data.dat  mode=Lazy  writesize=512  autorestart=off  dynamicfilemode=off  maxwritefilesize=512*1024^2
  scope1 : slrtlib/Displays and Logging/Scope   Commented=on  scopeno=5  scopetype=Target  autostart=on  viewmode=Graphical sliding  formatstr='%15.6f'  grid=on  ylimits=[0,400]  nosamples=30000  noprepostsamples=0  interleave=1  triggermode=FreeRun  triggersignal=1  trigsignalfromport=off  triggerlevel=0.0  triggerslope=Rising  triggerscope=1  triggersample=0  filename=data.dat  mode=Lazy  writesize=512  autorestart=off  dynamicfilemode=off  maxwritefilesize=512*1024^2
  scope2 : slrtlib/Displays and Logging/Scope   Commented=on  scopeno=6  scopetype=Target  autostart=on  viewmode=Graphical sliding  formatstr='%15.6f'  grid=on  ylimits=[0,40000]  nosamples=30000  noprepostsamples=0  interleave=1  triggermode=FreeRun  triggersignal=1  trigsignalfromport=off  triggerlevel=0.0  triggerslope=Rising  triggerscope=1  triggersample=0  filename=data.dat  mode=Lazy  writesize=512  autorestart=off  dynamicfilemode=off  maxwritefilesize=512*1024^2
  wires:
  [Encoder_Actual_Position] -> Gain4/1
  [DunkA_TPDO_DesiredCurrent] -> Moving Average/1
  [Joystick_LatCmd] -> Data Type Conversion15/1
  [Joystick_LongCmd] -> Data Type Conversion16/1
  Data Type Conversion5/1 -> Bus Creator2/1  "Encoder_Stored_Position"
  Bus Selector3/3 -> [AN_03]  "<Channel_AN3>"
  [DunkA_ActualCurrent] -> Data Type Conversion9/1
  [AN_01] -> Data Type Conversion17/1  "AN1"
  Bus Creator2/1 -> scope1/1
  Bus Selector1/2 -> [DunkA_ActualVelocity]  "<DunkA_ActualVelocity>"
  Data Type Conversion15/1 -> Joystick_LatCmd/1  "Joystick_LatCmd"
  Constant/1 -> [DunkA_TPDO_DesiredCurrent]
  [AN_04] -> Data Type Conversion21/1  "AN4"
  Data Type Conversion9/1 -> Bus Creator1/1  "Actual_Current"
  [DunkA_ActualVelocity] -> ActualVelocity/1  "DunkA_TPDO_ActualVelocity"
  Gain4/1 -> Data Type Conversion18/1
  Data Type Conversion19/1 -> Bus Creator3/2  "AN2"
  Joystick/1 -> Bus Selector8/1
  Bus Selector1/1 -> [DunkA_ActualCurrent]  "<DunkA_ActualCurrent>"
  Data Type Conversion18/1 -> Bus Creator2/2  "Encoder_Actual_Position"
  Data Type Conversion14/1 -> Bus Creator1/2  "Desired_Current"
  [Encoder_Stored_Position] -> Gain2/1
  Data Type Conversion20/1 -> Bus Creator3/3  "AN3"
  Moving Average/1 -> Data Type Conversion14/1
  Encoder/1 -> Bus Selector2/1
  Bus Selector8/1 -> [Joystick_LongCmd]  "<Joystick_LongCmd>"
  [AN_03] -> Data Type Conversion20/1  "AN3"
  Bus Selector8/2 -> [Joystick_LatCmd]  "<Joystick_LatCmd>"
  Bus Selector2/2 -> [Encoder_Actual_Position]  "<Encoder_Stored_Position>"
  Data Type Conversion16/1 -> Joystick_LongCmd/1  "Joystick_LongCmd"
  Bus Creator3/1 -> scope2/1
  [AN_02] -> Data Type Conversion19/1  "AN2"
  Data Type Conversion17/1 -> Bus Creator3/1  "AN1"
  Gain2/1 -> Data Type Conversion5/1
  Data Type Conversion21/1 -> Bus Creator3/4  "AN4"
  Bus Creator1/1 -> scope0/1
  Bus Selector3/2 -> [AN_02]  "<Channel_AN2>"
  Bus Selector3/1 -> [AN_01]  "<Channel_AN1>"
  Bus Selector2/1 -> [Encoder_Stored_Position]  "<Encoder_Actual_Position>"
  Bus Selector3/4 -> [AN_04]  "<Channel_AN4>"
  AN2CAN/1 -> Bus Selector3/1
  DunkA/1 -> Bus Selector1/1

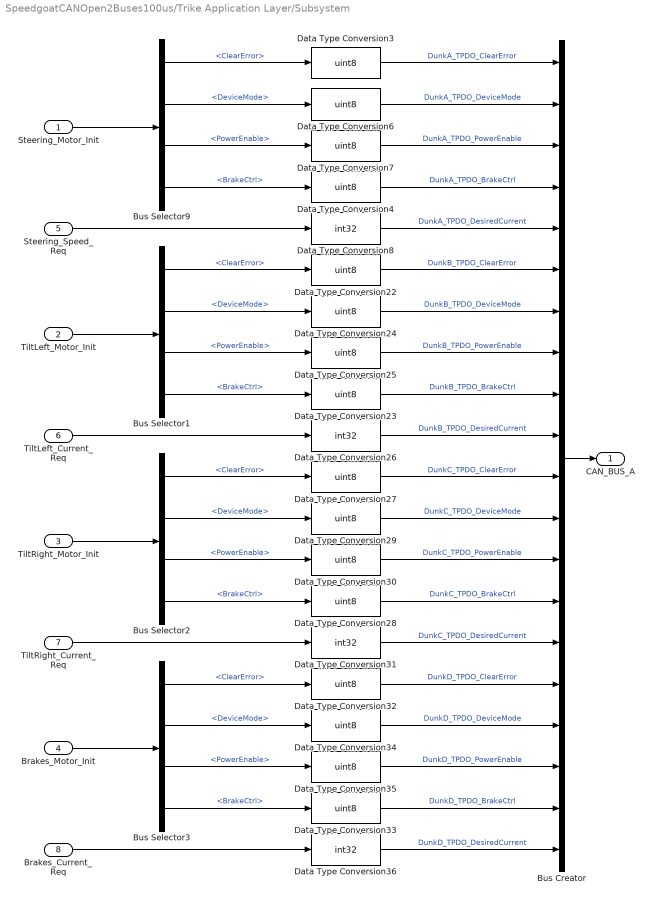
== system SpeedgoatCANOpen2Buses100us/Trike Application Layer/Subsystem ==
  Steering_Motor_Init : Inport  OutDataTypeStr=Bus: Dunk_Init_TPDOs
  TiltLeft_Motor_Init : Inport  Port=2  OutDataTypeStr=Bus: Dunk_Init_TPDOs
  TiltRight_Motor_Init : Inport  Port=3  OutDataTypeStr=Bus: Dunk_Init_TPDOs
  Brakes_Motor_Init : Inport  Port=4  OutDataTypeStr=Bus: Dunk_Init_TPDOs
  Steering_Speed_Req : Inport  Port=5
  TiltLeft_Current_Req : Inport  Port=6
  TiltRight_Current_Req : Inport  Port=7
  Brakes_Current_Req : Inport  Port=8
  Bus Creator : BusCreator  Inputs=20  OutDataTypeStr=Bus: CAN_BUS_A
  Bus Selector{1..3,9} (4 alike) : BusSelector  OutputSignals=ClearError,DeviceMode,PowerEnable,BrakeCtrl
  Data Type Conversion{3..4,6..7,22..25,27..30,32..35} (16 alike) : DataTypeConversion  OutDataTypeStr=uint8
  Data Type Conversion{8,26,31,36} (4 alike) : DataTypeConversion  OutDataTypeStr=int32
  CAN_BUS_A : Outport  OutDataTypeStr=Bus: CAN_BUS_A
  wires:
  Data Type Conversion31/1 -> Bus Creator/15  "DunkC_TPDO_DesiredCurrent"
  Data Type Conversion34/1 -> Bus Creator/17  "DunkD_TPDO_DeviceMode"
  Data Type Conversion32/1 -> Bus Creator/16  "DunkD_TPDO_ClearError"
  Data Type Conversion23/1 -> Bus Creator/9  "DunkB_TPDO_BrakeCtrl"
  Data Type Conversion25/1 -> Bus Creator/8  "DunkB_TPDO_PowerEnable"
  Data Type Conversion36/1 -> Bus Creator/20  "DunkD_TPDO_DesiredCurrent"
  Data Type Conversion6/1 -> Bus Creator/2  "DunkA_TPDO_DeviceMode"
  Data Type Conversion26/1 -> Bus Creator/10  "DunkB_TPDO_DesiredCurrent"
  Data Type Conversion30/1 -> Bus Creator/13  "DunkC_TPDO_PowerEnable"
  Data Type Conversion28/1 -> Bus Creator/14  "DunkC_TPDO_BrakeCtrl"
  Data Type Conversion27/1 -> Bus Creator/11  "DunkC_TPDO_ClearError"
  Data Type Conversion24/1 -> Bus Creator/7  "DunkB_TPDO_DeviceMode"
  Bus Creator/1 -> CAN_BUS_A/1
  Data Type Conversion29/1 -> Bus Creator/12  "DunkC_TPDO_DeviceMode"
  Data Type Conversion33/1 -> Bus Creator/19  "DunkD_TPDO_BrakeCtrl"
  Data Type Conversion35/1 -> Bus Creator/18  "DunkD_TPDO_PowerEnable"
  Data Type Conversion22/1 -> Bus Creator/6  "DunkB_TPDO_ClearError"
  Data Type Conversion4/1 -> Bus Creator/4  "DunkA_TPDO_BrakeCtrl"
  Data Type Conversion3/1 -> Bus Creator/1  "DunkA_TPDO_ClearError"
  Data Type Conversion8/1 -> Bus Creator/5  "DunkA_TPDO_DesiredCurrent"
  Data Type Conversion7/1 -> Bus Creator/3  "DunkA_TPDO_PowerEnable"
  Steering_Motor_Init/1 -> Bus Selector9/1
  Bus Selector9/1 -> Data Type Conversion3/1  "<ClearError>"
  Bus Selector9/2 -> Data Type Conversion6/1  "<DeviceMode>"
  Bus Selector9/3 -> Data Type Conversion7/1  "<PowerEnable>"
  Bus Selector9/4 -> Data Type Conversion4/1  "<BrakeCtrl>"
  Steering_Speed_Req/1 -> Data Type Conversion8/1
  Bus Selector1/1 -> Data Type Conversion22/1  "<ClearError>"
  Bus Selector1/2 -> Data Type Conversion24/1  "<DeviceMode>"
  Bus Selector1/3 -> Data Type Conversion25/1  "<PowerEnable>"
  Bus Selector1/4 -> Data Type Conversion23/1  "<BrakeCtrl>"
  TiltLeft_Current_Req/1 -> Data Type Conversion26/1
  TiltLeft_Motor_Init/1 -> Bus Selector1/1
  Bus Selector2/1 -> Data Type Conversion27/1  "<ClearError>"
  Bus Selector2/2 -> Data Type Conversion29/1  "<DeviceMode>"
  Bus Selector2/3 -> Data Type Conversion30/1  "<PowerEnable>"
  Bus Selector2/4 -> Data Type Conversion28/1  "<BrakeCtrl>"
  Bus Selector3/1 -> Data Type Conversion32/1  "<ClearError>"
  Bus Selector3/2 -> Data Type Conversion34/1  "<DeviceMode>"
  TiltRight_Current_Req/1 -> Data Type Conversion31/1
  Brakes_Current_Req/1 -> Data Type Conversion36/1
  TiltRight_Motor_Init/1 -> Bus Selector2/1
  Brakes_Motor_Init/1 -> Bus Selector3/1
  Bus Selector3/3 -> Data Type Conversion35/1  "<PowerEnable>"
  Bus Selector3/4 -> Data Type Conversion33/1  "<BrakeCtrl>"

== system SpeedgoatCANOpen2Buses100us/Trike Application Layer/Subsystem1 ==
  APT_ControlWord : Inport
  APT_PedalPosition : Inport  Port=2
  Bus Creator : BusCreator  Inputs=3  OutDataTypeStr=Bus: CAN_BUS_B
  Data Type Conversion : DataTypeConversion  OutDataTypeStr=uint8
  Data Type Conversion1 : DataTypeConversion  OutDataTypeStr=uint8
  Data Type Conversion2 : DataTypeConversion  OutDataTypeStr=uint8
  HeartBeatgenerator : MATLAB Function  TreatAsAtomicUnit=on
  CAN_BUS_B : Outport  OutDataTypeStr=Bus: CAN_BUS_B
  wires:
  Bus Creator/1 -> CAN_BUS_B/1
  APT_ControlWord/1 -> Data Type Conversion/1
  Data Type Conversion2/1 -> Bus Creator/3  "APT_TPDO_Heartbeat"
  APT_PedalPosition/1 -> Data Type Conversion1/1
  HeartBeatgenerator/1(HB) -> Data Type Conversion2/1
  Data Type Conversion1/1 -> Bus Creator/2  "APT_TPDO_PedalPosition"
  Data Type Conversion/1 -> Bus Creator/1  "APT_TPDO_ControlWord"

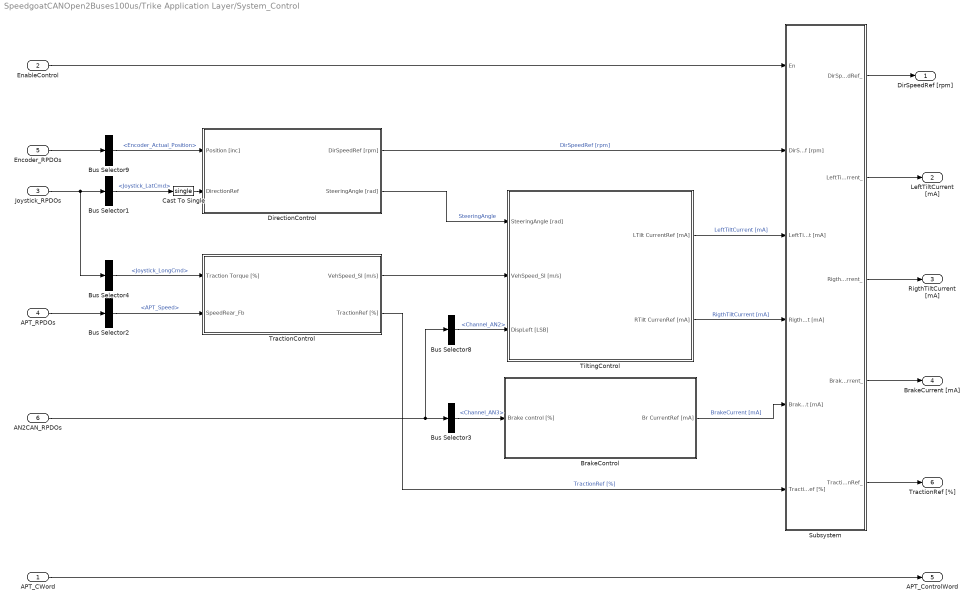
== system SpeedgoatCANOpen2Buses100us/Trike Application Layer/System_Control ==
  APT_CWord : Inport
  EnableControl : Inport  Port=2
  Joystick_RPDOs : Inport  Port=3  OutDataTypeStr=Bus: Joystick_RPDOs
  APT_RPDOs : Inport  Port=4  OutDataTypeStr=Bus: APT_RPDOs
  Encoder_RPDOs : Inport  Port=5  OutDataTypeStr=Bus: Encoder_RPDOs
  AN2CAN_RPDOs : Inport  Port=6  OutDataTypeStr=Bus: AN2CAN_conv
  BrakeControl : Subsystem
  Bus Selector1 : BusSelector  OutputSignals=Joystick_LatCmd
  Bus Selector2 : BusSelector  OutputSignals=APT_Speed
  Bus Selector3 : BusSelector  OutputSignals=Channel_AN3
  Bus Selector4 : BusSelector  OutputSignals=Joystick_LongCmd
  Bus Selector8 : BusSelector  OutputSignals=Channel_AN2
  Bus Selector9 : BusSelector  OutputSignals=Encoder_Actual_Position
  Cast To Single : DataTypeConversion  OutDataTypeStr=single
  DirectionControl : Subsystem
  Subsystem : Subsystem
  TiltingControl : Subsystem
  TractionControl : Subsystem
  DirSpeedRef [rpm] : Outport
  LeftTiltCurrent [mA] : Outport  Port=2
  RigthTiltCurrent [mA] : Outport  Port=3
  BrakeCurrent [mA] : Outport  Port=4
  APT_ControlWord : Outport  Port=5
  TractionRef [%] : Outport  Port=6
  wires:
  Bus Selector1/1 -> Cast To Single/1  "<Joystick_LatCmd>"
  DirectionControl/2(SteeringAngle [rad]) -> TiltingControl/1(SteeringAngle [rad])  "SteeringAngle"
  Bus Selector4/1 -> TractionControl/1(Traction Torque [%])  "<Joystick_LongCmd>"
  Bus Selector2/1 -> TractionControl/2(SpeedRear_Fb)  "<APT_Speed>"
  TractionControl/1(VehSpeed_SI [m/s]) -> TiltingControl/2(VehSpeed_SI [m/s])
  Encoder_RPDOs/1 -> Bus Selector9/1
  AN2CAN_RPDOs/1 -> Bus Selector3/1, Bus Selector8/1
  Bus Selector8/1 -> TiltingControl/3(DispLeft [LSB])  "<Channel_AN2>"
  Bus Selector9/1 -> DirectionControl/1(Position [inc])  "<Encoder_Actual_Position>"
  APT_RPDOs/1 -> Bus Selector2/1
  Joystick_RPDOs/1 -> Bus Selector4/1, Bus Selector1/1
  Bus Selector3/1 -> BrakeControl/1(Brake control [%])  "<Channel_AN3>"
  EnableControl/1 -> Subsystem/1(En)
  DirectionControl/1(DirSpeedRef [rpm]) -> Subsystem/2(DirSpeedRef [rpm])  "DirSpeedRef [rpm]"
  TiltingControl/1(LTilt CurrentRef [mA]) -> Subsystem/3(LeftTiltCurrent [mA])  "LeftTiltCurrent [mA]"
  TractionControl/2(TractionRef [%]) -> Subsystem/6(TractionRef [%])  "TractionRef [%]"
  TiltingControl/2(RTilt CurrenRef [mA]) -> Subsystem/4(RigthTiltCurrent [mA])  "RigthTiltCurrent [mA]"
  BrakeControl/1(Br CurrentRef [mA]) -> Subsystem/5(BrakeCurrent [mA])  "BrakeCurrent [mA]"
  Subsystem/1(DirSpeedRef_) -> DirSpeedRef [rpm]/1
  Subsystem/2(LeftTiltCurrent_) -> LeftTiltCurrent [mA]/1
  Subsystem/3(RigthTiltCurrent_) -> RigthTiltCurrent [mA]/1
  Subsystem/4(BrakeCurrent_) -> BrakeCurrent [mA]/1
  Subsystem/5(TractionRef_) -> TractionRef [%]/1
  Cast To Single/1 -> DirectionControl/2(DirectionRef)
  APT_CWord/1 -> APT_ControlWord/1

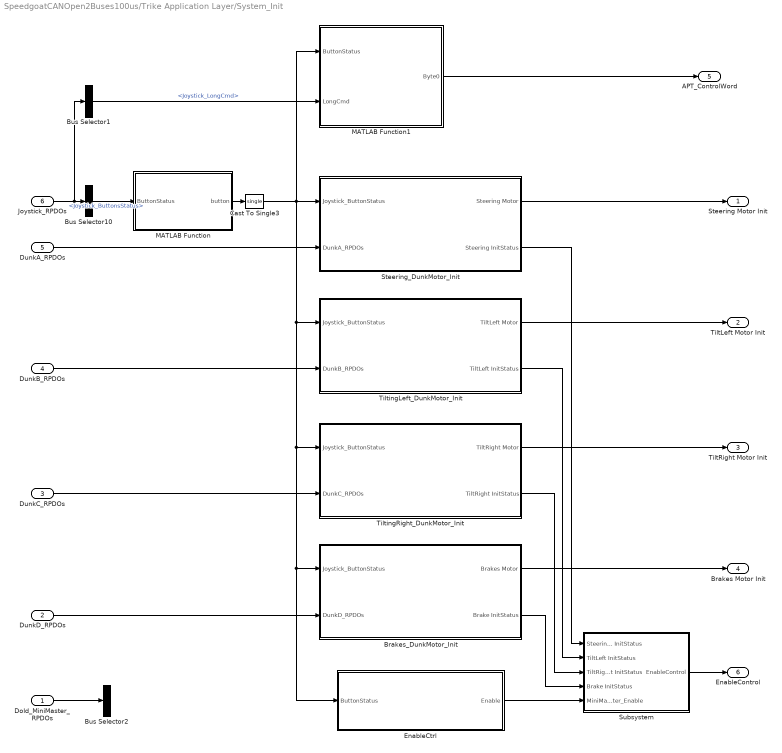
== system SpeedgoatCANOpen2Buses100us/Trike Application Layer/System_Init ==
  Dold_MiniMaster_RPDOs : Inport  OutDataTypeStr=Bus: Dold_RPDOs
  DunkD_RPDOs : Inport  Port=2  OutDataTypeStr=Bus: Dunk_RPDOs
  DunkC_RPDOs : Inport  Port=3  OutDataTypeStr=Bus: Dunk_RPDOs
  DunkB_RPDOs : Inport  Port=4  OutDataTypeStr=Bus: Dunk_RPDOs
  DunkA_RPDOs : Inport  Port=5  OutDataTypeStr=Bus: Dunk_RPDOs
  Joystick_RPDOs : Inport  Port=6  OutDataTypeStr=Bus: Joystick_RPDOs
  Brakes_DunkMotor_Init : Subsystem
  Bus Selector1 : BusSelector  OutputSignals=Joystick_LongCmd
  Bus Selector10 : BusSelector  OutputSignals=Joystick_ButtonsStatus
  Bus Selector2 : BusSelector  OutputSignals=Enable
  Cast To Single3 : DataTypeConversion  OutDataTypeStr=single
  EnableCtrl : Stateflow chart  TreatAsAtomicUnit=on
  MATLAB Function : MATLAB Function  TreatAsAtomicUnit=on
  MATLAB Function1 : MATLAB Function  TreatAsAtomicUnit=on
  Steering_DunkMotor_Init : Subsystem
  Subsystem : Subsystem
  TiltingLeft_DunkMotor_Init : Subsystem
  TiltingRight_DunkMotor_Init : Subsystem
  Steering Motor Init : Outport  OutDataTypeStr=Bus: Dunk_Init_TPDOs
  TiltLeft Motor Init : Outport  Port=2  OutDataTypeStr=Bus: Dunk_Init_TPDOs
  TiltRight Motor Init : Outport  Port=3  OutDataTypeStr=Bus: Dunk_Init_TPDOs
  Brakes Motor Init : Outport  Port=4  OutDataTypeStr=Bus: Dunk_Init_TPDOs
  APT_ControlWord : Outport  Port=5
  EnableControl : Outport  Port=6
  wires:
  Bus Selector10/1 -> MATLAB Function/1(ButtonStatus)  "<Joystick_ButtonsStatus>"
  Joystick_RPDOs/1 -> Bus Selector1/1, Bus Selector10/1
  DunkD_RPDOs/1 -> Brakes_DunkMotor_Init/2(DunkD_RPDOs)
  DunkC_RPDOs/1 -> TiltingRight_DunkMotor_Init/2(DunkC_RPDOs)
  DunkB_RPDOs/1 -> TiltingLeft_DunkMotor_Init/2(DunkB_RPDOs)
  DunkA_RPDOs/1 -> Steering_DunkMotor_Init/2(DunkA_RPDOs)
  Steering_DunkMotor_Init/1(Steering Motor) -> Steering Motor Init/1
  TiltingLeft_DunkMotor_Init/1(TiltLeft Motor) -> TiltLeft Motor Init/1
  TiltingRight_DunkMotor_Init/1(TiltRight Motor) -> TiltRight Motor Init/1
  Brakes_DunkMotor_Init/1(Brakes Motor) -> Brakes Motor Init/1
  MATLAB Function1/1(Byte0) -> APT_ControlWord/1
  Bus Selector1/1 -> MATLAB Function1/2(LongCmd)  "<Joystick_LongCmd>"
  MATLAB Function/1(button) -> Cast To Single3/1
  Cast To Single3/1 -> EnableCtrl/1(ButtonStatus), Brakes_DunkMotor_Init/1(Joystick_ButtonStatus), TiltingRight_DunkMotor_Init/1(Joystick_ButtonStatus), TiltingLeft_DunkMotor_Init/1(Joystick_ButtonStatus), MATLAB Function1/1(ButtonStatus), Steering_DunkMotor_Init/1(Joystick_ButtonStatus)
  Steering_DunkMotor_Init/2(Steering InitStatus) -> Subsystem/1(Steering InitStatus)
  TiltingLeft_DunkMotor_Init/2(TiltLeft InitStatus) -> Subsystem/2(TiltLeft InitStatus)
  TiltingRight_DunkMotor_Init/2(TiltRight InitStatus) -> Subsystem/3(TiltRight InitStatus)
  Brakes_DunkMotor_Init/2(Brake InitStatus) -> Subsystem/4(Brake InitStatus)
  Subsystem/1(EnableControl) -> EnableControl/1
  Dold_MiniMaster_RPDOs/1 -> Bus Selector2/1
  EnableCtrl/1(Enable) -> Subsystem/5(MiniMaster_Enable)

== system SpeedgoatCANOpen2Buses100us/Speedgoat_TPDOs/CAN Bus Communication/CANOpen Slave Protocol Stack - CAN Bus #1 (A) ==
  C Caller : CCaller  FunctionName=CANOpenSlave_ProcessStack  PortSpecificationStruct="%)30     .    ( D   8    (     @         %    \"     8    !     0         %  0 \"0    $    V    07)G3F%M90  4&]R=$YA;64 4V-O<&4     26YD97@     5'EP90      4VEZ90         .    ,     8    (    !          %    \"     $    $     0         0  0 <GA)1 X    P    !@    @    $          4    (     0    0    !         !  ! !R>$E$#@   #@    &    \"     0         !0    @    !    !0    $         $     4   !);G ...(+2763 chars)"
  CAN RX Wrapper : Subsystem
  CAN TX Wrapper : Subsystem
  wires:
  C Caller/2 -> CAN TX Wrapper/Enable, CAN TX Wrapper/2(DLC)
  CAN RX Wrapper/1(ID) -> C Caller/1
  C Caller/1 -> CAN TX Wrapper/1(ID)
  CAN RX Wrapper/2(DLC) -> C Caller/2
  C Caller/3 -> CAN TX Wrapper/3(DATA)
  CAN RX Wrapper/3(DATA) -> C Caller/3
